simulink model "sub3"  (Simulink 6.0)
settings: Solver=ode5  StartTime=0.0  StopTime=10.0  RelTol=1e-3
undefined symbols (not defined in the file): dkd, dki, dkp
settings Model: LastModifiedBy=Administrator

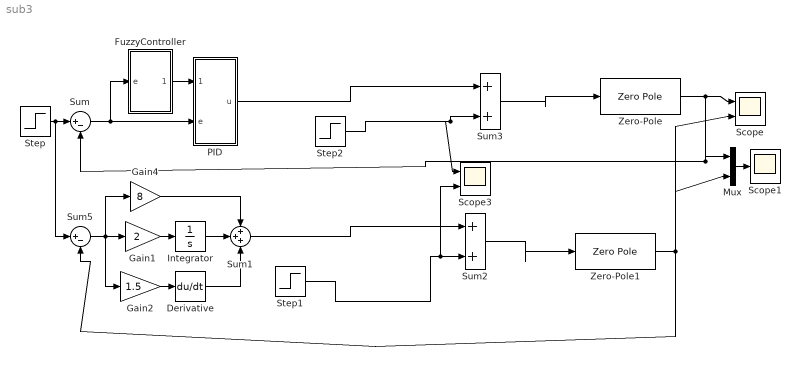
== system sub3 ==
  Derivative : Derivative
  FuzzyController : Subsystem
  Gain1 : Gain  Gain=2
  Gain2 : Gain  Gain=1.5
  Gain4 : Gain  Gain=8
  Integrator : Integrator
  Mux : Mux  Inputs=2
  PID : Subsystem
  Scope : Scope  NumInputPorts=2
      settings: TimeRange=20  YMin=1.00028~0.99525  YMax=1.00031~0.99555
  Scope1 : Scope
      settings: TimeRange=10  YMin=0.86  YMax=1.04  SaveName=ScopeData2
  Scope3 : Scope  NumInputPorts=2
      settings: TimeRange=20  YMin=1.00028~0.99525  YMax=1.00031~0.99555  SaveName=ScopeData4
  Step : Step  Time=0  SampleTime=0
  Step1 : Step  Time=4  SampleTime=0
  Step2 : Step  Time=4  SampleTime=0
  Sum : Sum  Inputs=|+-
  Sum1 : Sum  Inputs=+++
  Sum2 : Sum  Inputs=|++
  Sum3 : Sum  Inputs=|++
  Sum5 : Sum  Inputs=|+-
  Zero-Pole : ZeroPole  Zeros=[-0.5]  Poles=[-1 -1 -1]  Gain=[10]
  Zero-Pole1 : ZeroPole  Zeros=[-0.5]  Poles="[-1  -1 -1]"  Gain=[10]
  wires:
  Step/1 -> Sum/1, Sum5/1
  Sum/1 -> PID/2(e), FuzzyController/1(e)
  Zero-Pole/1 -> Scope/1, Sum/2, Mux/1
  FuzzyController/1(dPID) -> PID/1(dPID)
  Sum5/1 -> Gain1/1, Gain2/1, Gain4/1
  Gain2/1 -> Derivative/1
  Gain1/1 -> Integrator/1
  Integrator/1 -> Sum1/2
  Derivative/1 -> Sum1/3
  Zero-Pole1/1 -> Sum5/2, Scope/2, Mux/2
  Gain4/1 -> Sum1/1
  Mux/1 -> Scope1/1
  Sum1/1 -> Sum2/1
  PID/1(u) -> Sum3/1
  Sum2/1 -> Zero-Pole1/1
  Sum3/1 -> Zero-Pole/1
  Step1/1 -> Sum2/2, Scope3/2
  Step2/1 -> Sum3/2, Scope3/1

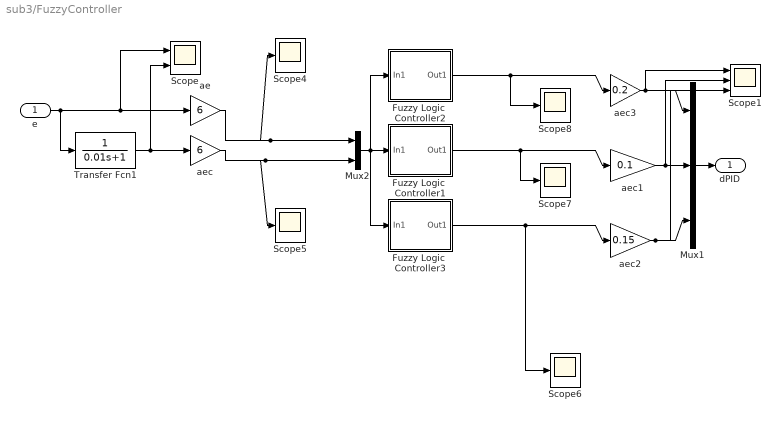
== system sub3/FuzzyController ==
  e : Inport  Port=1  LatchInput=off
  Fuzzy Logic  Controller1 : Subsystem  AncestorBlock="fuzblock/Fuzzy Logic  Controller"  mask(FIS){fis=dki}
      mask prompts: fis "FIS File or Structure:"
      mask help: FIS
      mask init:
      | fis = fuzblockmask(gcb,fis);
      mask Help: web(['file:///' docroot '/toolbox/fuzzy/fuzzylogiccontroller.html']);
      mask Display: plot(0, -0.3, 6, -0.3, 0, 1.2, 6, 1.2, [0 6], [0 0], [1 2 3],[0 1 0],[2 3 4],[0 1 0],[3 4 5],[0 1 0])
  Fuzzy Logic  Controller2 : Subsystem  AncestorBlock="fuzblock/Fuzzy Logic  Controller"  mask(FIS){fis=dkp}
      mask prompts: fis "FIS File or Structure:"
      mask help: FIS
      mask init:
      | fis = fuzblockmask(gcb,fis);
      mask Help: web(['file:///' docroot '/toolbox/fuzzy/fuzzylogiccontroller.html']);
      mask Display: plot(0, -0.3, 6, -0.3, 0, 1.2, 6, 1.2, [0 6], [0 0], [1 2 3],[0 1 0],[2 3 4],[0 1 0],[3 4 5],[0 1 0])
  Fuzzy Logic  Controller3 : Subsystem  AncestorBlock="fuzblock/Fuzzy Logic  Controller"  mask(FIS){fis=dkd}
      mask prompts: fis "FIS File or Structure:"
      mask help: FIS
      mask init:
      | fis = fuzblockmask(gcb,fis);
      mask Help: web(['file:///' docroot '/toolbox/fuzzy/fuzzylogiccontroller.html']);
      mask Display: plot(0, -0.3, 6, -0.3, 0, 1.2, 6, 1.2, [0 6], [0 0], [1 2 3],[0 1 0],[2 3 4],[0 1 0],[3 4 5],[0 1 0])
  Mux1 : Mux  Inputs=3
  Mux2 : Mux  Inputs=2
  Scope : Scope  NumInputPorts=2
      settings: TimeRange=10  YMin=-0.0115~-0.012  YMax=-0.0015~-0.0015  SaveName=ScopeData10
  Scope1 : Scope  NumInputPorts=3
      settings: TimeRange=10  YMin=-1~-0.5~-0.5  YMax=1~0.5~0.5
  Scope{4..8} (5 alike) : Scope
      Scope4 settings: TimeRange=10  YMin=0.2  YMax=1.3  SaveName=ScopeData5
      Scope5 settings: TimeRange=10  YMin=0.2  YMax=1.3  SaveName=ScopeData6
      Scope6 settings: TimeRange=10  YMin=0.2  YMax=1.3  SaveName=ScopeData7
      Scope7 settings: TimeRange=10  YMin=0.2  YMax=1.3  SaveName=ScopeData8
      Scope8 settings: TimeRange=10  YMin=0.2  YMax=1.3  SaveName=ScopeData9
  Transfer Fcn1 : TransferFcn  Denominator=[0.01 1]
  ae : Gain  Gain=6
  aec : Gain  Gain=6
  aec1 : Gain  Gain=0.1
  aec2 : Gain  Gain=0.15
  aec3 : Gain  Gain=0.2
  dPID : Outport  OutDataType=fixdt(1,16,0)  OutScaling=[]
  wires:
  Fuzzy Logic  Controller2/1(Out1) -> aec3/1, Scope8/1
  Fuzzy Logic  Controller1/1(Out1) -> aec1/1, Scope7/1
  Fuzzy Logic  Controller3/1(Out1) -> aec2/1, Scope6/1
  e/1 -> Transfer Fcn1/1, ae/1, Scope/1
  Transfer Fcn1/1 -> aec/1, Scope/2
  ae/1 -> Mux2/1, Scope4/1
  aec/1 -> Mux2/2, Scope5/1
  Mux2/1 -> Fuzzy Logic  Controller1/1(In1), Fuzzy Logic  Controller3/1(In1), Fuzzy Logic  Controller2/1(In1)
  aec1/1 -> Mux1/2, Scope1/2
  aec2/1 -> Mux1/3, Scope1/3
  aec3/1 -> Mux1/1, Scope1/1
  Mux1/1 -> dPID/1

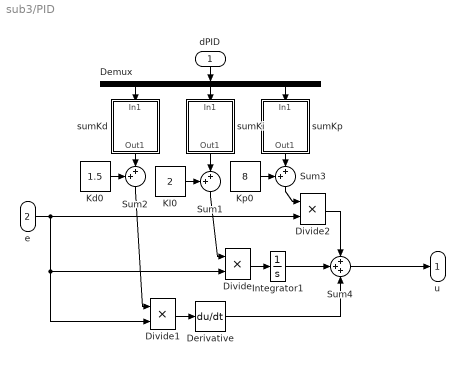
== system sub3/PID ==
  dPID : Inport  Orientation=down  Port=1  OutDataType=fixdt(1,16,0)  OutScaling=[]  LatchInput=off
  e : Inport  Port=2  OutDataType=fixdt(1,16,0)  OutScaling=[]  LatchInput=off
  Demux : Demux  Orientation=down  Outputs=3
  Derivative : Derivative
  Divide : Product  Inputs=**  OutScaling=2^-10
  Divide1 : Product  Inputs=**  OutScaling=2^-10
  Divide2 : Product  Inputs=**  OutScaling=2^-10
  Integrator1 : Integrator
  KI0 : Constant  Value=2
  Kd0 : Constant  Value=1.5
  Kp0 : Constant  Value=8
  Sum1 : Sum  Orientation=down  Inputs=++|
  Sum2 : Sum  Orientation=down  Inputs=++|
  Sum3 : Sum  Orientation=down  Inputs=++|
  Sum4 : Sum  Inputs=+++
  sumKd : Subsystem  Orientation=down
  sumKi : Subsystem  Orientation=down
  sumKp : Subsystem  Orientation=down
  u : Outport
  wires:
  Sum3/1 -> Divide2/1
  Sum2/1 -> Divide1/1
  Kp0/1 -> Sum3/1
  Kd0/1 -> Sum2/1
  KI0/1 -> Sum1/1
  Sum1/1 -> Divide/1
  e/1 -> Divide2/2, Divide/2, Divide1/2
  Divide2/1 -> Sum4/1
  Divide/1 -> Integrator1/1
  Divide1/1 -> Derivative/1
  Sum4/1 -> u/1
  dPID/1 -> Demux/1
  Demux/3 -> sumKp/1(In1)
  Demux/2 -> sumKi/1(In1)
  Demux/1 -> sumKd/1(In1)
  Integrator1/1 -> Sum4/2
  Derivative/1 -> Sum4/3
  sumKp/1(Out1) -> Sum3/2
  sumKi/1(Out1) -> Sum1/2
  sumKd/1(Out1) -> Sum2/2

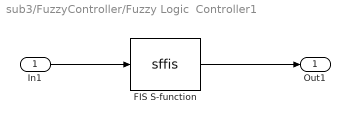
== system sub3/FuzzyController/Fuzzy Logic  Controller1 ==
  In1 : Inport  Port=1  LatchInput=off
  FIS S-function : S-Function  FunctionName=sffis  Parameters=fis  SFunctionModules=sfsup
  Out1 : Outport
  wires:
  FIS S-function/1 -> Out1/1
  In1/1 -> FIS S-function/1

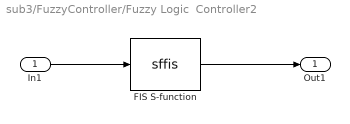
== system sub3/FuzzyController/Fuzzy Logic  Controller2 ==
  In1 : Inport  Port=1  LatchInput=off
  FIS S-function : S-Function  FunctionName=sffis  Parameters=fis  SFunctionModules=sfsup
  Out1 : Outport
  wires:
  In1/1 -> FIS S-function/1
  FIS S-function/1 -> Out1/1

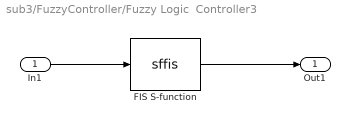
== system sub3/FuzzyController/Fuzzy Logic  Controller3 ==
  In1 : Inport  Port=1  LatchInput=off
  FIS S-function : S-Function  FunctionName=sffis  Parameters=fis  SFunctionModules=sfsup
  Out1 : Outport
  wires:
  In1/1 -> FIS S-function/1
  FIS S-function/1 -> Out1/1

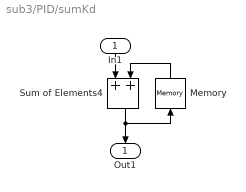
== system sub3/PID/sumKd ==
  In1 : Inport  Orientation=down  Port=1  OutDataType=fixdt(1,16,0)  OutScaling=[]  LatchInput=off
  Memory : Memory  Orientation=up  InheritSampleTime=on
  Sum of Elements4 : Sum  Orientation=down  OutScaling=2^-10  SampleTime=0.001
  Out1 : Outport  Orientation=down  OutDataType=fixdt(1,16,0)  OutScaling=[]
  wires:
  Sum of Elements4/1 -> Out1/1, Memory/1
  Memory/1 -> Sum of Elements4/2
  In1/1 -> Sum of Elements4/1

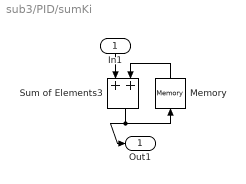
== system sub3/PID/sumKi ==
  In1 : Inport  Orientation=down  Port=1  OutDataType=fixdt(1,16,0)  OutScaling=[]  LatchInput=off
  Memory : Memory  Orientation=up  InheritSampleTime=on
  Sum of Elements3 : Sum  Orientation=down  OutScaling=2^-10  SampleTime=0.001
  Out1 : Outport  OutDataType=fixdt(1,16,0)  OutScaling=[]
  wires:
  Sum of Elements3/1 -> Out1/1, Memory/1
  Memory/1 -> Sum of Elements3/2
  In1/1 -> Sum of Elements3/1

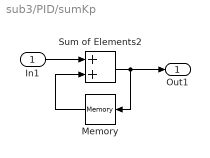
== system sub3/PID/sumKp ==
  In1 : Inport  Port=1  OutDataType=fixdt(1,16,0)  OutScaling=[]  LatchInput=off
  Memory : Memory  Orientation=left  InheritSampleTime=on
  Sum of Elements2 : Sum  OutScaling=2^-10  SampleTime=0.001
  Out1 : Outport  OutDataType=fixdt(1,16,0)  OutScaling=[]
  wires:
  In1/1 -> Sum of Elements2/1
  Memory/1 -> Sum of Elements2/2
  Sum of Elements2/1 -> Out1/1, Memory/1
